simulink model "WDS"  (R2022a)
settings: Solver=FixedStepDiscrete  StartTime=0.0  StopTime=T_final  FixedStep=T_sample  RelTol=1e-3
values from neighbouring files (symbols this model uses):
  A_bar_d = readmatrix('A_bar_d.csv')    [Run_model.m]    (also in prepare_trajectory_data.m = [0.9950 0.0998)
  B_bar_d = readmatrix('B_bar_d.csv')    [Run_model.m]    (also in prepare_trajectory_data.m = [0.1)
  C_obsv_d = [-0.48244804282  -0.463279461508; 0.0144227342104  -0.230554726046; 0.244765695792  -0.329721244669; 0.487562807757  0.730038636795; 0.684075320502  -0.191202440855; 0.0380669049625  0.232348391545]    [C_obsv_d.mat]    (also in Run_model.m = readmatrix('C_obsv_d.csv'); sys_generation_WDS.m = C_obsv)
  Cm = ones(1,n_states)    [Run_model.m]
  D_obsv_d = readmatrix('D_obsv_d.csv')    [Run_model.m]    (also in prepare_trajectory_data.m = zeros(n_meas,n_int); sys_generation_WDS.m = D_obsv)
  x0 = 0.3+ 0.2*rand(n_states,1)    [Run_model.m]    (also in prepare_trajectory_data.m = [7;7]; test.m = rand(n_states,1))
settings Model: Creator=Abelb  LastModifiedBy=Abelb
settings DebuggingCC: UnconnectedInputMsg=warning  UnconnectedOutputMsg=warning  UnconnectedLineMsg=warning
settings RTWCC: DLArmComputeVersion=19.05

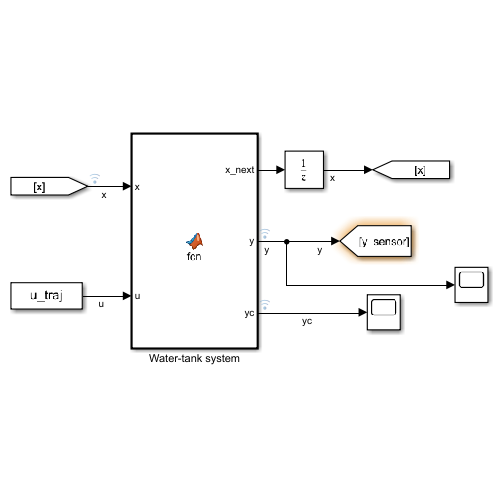
[thumbnail: Simulink's stored preview of the top-level diagram]
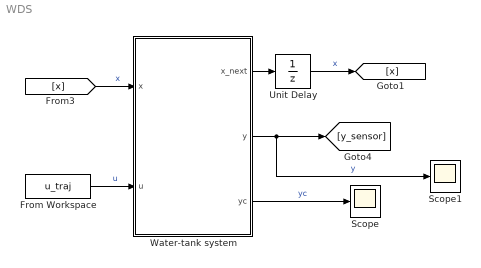
== system WDS ==
  From Workspace : FromWorkspace  VariableName=u_traj
  Scope : Scope
  Scope1 : Scope
  Unit Delay : UnitDelay  InitialCondition=x0  SampleTime=-1  HasFrameUpgradeWarning=on
  Water-tank system : MATLAB Function  TreatAsAtomicUnit=on
  wires:
  Water-tank system/1(x_next) -> Unit Delay/1
  From Workspace/1 -> Water-tank system/2(u)  "u"
  Water-tank system/2(y) -> Scope1/1, [y_sensor]  "y"
  Water-tank system/3(yc) -> Scope/1  "yc"
  Unit Delay/1 -> [x]  "x"
  [x] -> Water-tank system/1(x)  "x"

== matlab function WDS/Water-tank system ==
  data: x input; x_next output; u input; y output; A_bar_d parameter; C_obsv_d parameter; B_bar_d parameter; D_obsv_d parameter; Cm parameter; yc output
function [x_next,y,yc] = fcn(x,u,A_bar_d,C_obsv_d,B_bar_d,D_obsv_d,Cm)
% Discrete state-space model for system

x_next = A_bar_d*x + B_bar_d*u;

y = C_obsv_d*x + D_obsv_d*u;

% critical measurements
yc = Cm*x;
